simulink model "Main"  (R2020b)
settings: Solver=FixedStepAuto  StartTime=0.0  StopTime=10  FixedStep=0.01  RelTol=1e-3
libraries: TcSimInterface x1
(part 2 of 2)

== matlab function Main/Decode ==
  data: PlcToModel input; velocity output
function velocity  = DecodePlcMessage(PlcToModel)


velocity = bitand(PlcToModel, uint32(0xffff));

end

== matlab function Main/Encode ==
  data: counterValue input; modelToPlc output; driveState input
function modelToPlc = EncodePlcMessage(counterValue, driveState)
    modelToPlc = uint32(0);
    modelToPlc = bitor(modelToPlc, uint32(driveState));
    modelToPlc = bitshift(modelToPlc,16);
    
    modelToPlc = bitor(modelToPlc, uint32(counterValue));
    
    %modelToPlc = bitand(modelToPlc, bitshift(driveState,16));
    %modelToPlc = bitand(modelToPlc, counterValue);

end
